simulink model "Simulation_Angle_To_Servo"  (R2020a)
settings: Solver=VariableStepAuto  StartTime=0.0  StopTime=10.0  RelTol=1e-3
values from neighbouring files (symbols this model uses):
  AValues = griddata(data.alpha,data.beta,data.AngleservoA,Alpha,Beta)    [dataToLookupTable.m]
  BValues = griddata(data.alpha,data.beta,data.AngleservoB,Alpha,Beta)    [dataToLookupTable.m]
  CValues = griddata(data.alpha,data.beta,data.AngleservoC,Alpha,Beta)    [dataToLookupTable.m]
settings Model: Creator=vince  LastModifiedBy=vince

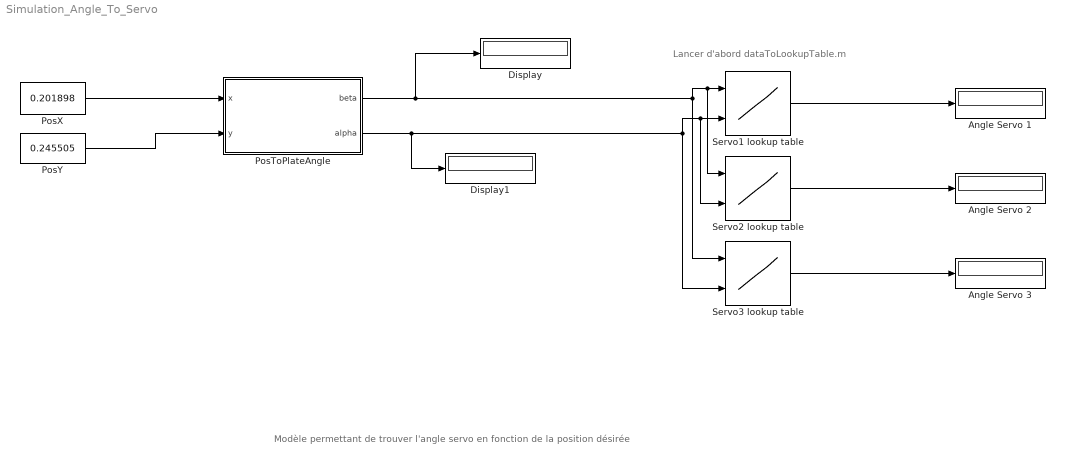
== system Simulation_Angle_To_Servo ==
  note: Modèle permettant de trouver l'angle servo en fonction de la position désirée
  note: Lancer d'abord dataToLookupTable.m
  Angle Servo 1 : Display
  Angle Servo 2 : Display
  Angle Servo 3 : Display
  Display : Display
  Display1 : Display
  PosToPlateAngle : MATLAB Function  TreatAsAtomicUnit=on
  PosX : Constant  Value=0.201898
  PosY : Constant  Value=0.245505
  Servo1 lookup table : Lookup_n-D  BreakpointsSpecification=Even spacing  BreakpointsForDimension1=[1:1801]  BreakpointsForDimension2=[1:176]  BreakpointsForDimension3=[2:316988]  BreakpointsForDimension1FirstPoint=0  BreakpointsForDimension2FirstPoint=0  BreakpointsForDimension1Spacing=0.2  BreakpointsForDimension2Spacing=0.2  IndexSearchMethod=Evenly spaced points  Table=AValues  TableDataTypeStr=Inherit: Inherit from 'Table data'  InterpMethod=Nearest  InternalRulePriority=Speed  OutMin=[3]  OutMax=[3]  OutDataTypeStr=Inherit: Inherit from 'Table data'  RndMeth=Simplest  InputSameDT=on
  Servo2 lookup table : Lookup_n-D  BreakpointsSpecification=Even spacing  BreakpointsForDimension1=[1:1801]  BreakpointsForDimension2=[1:176]  BreakpointsForDimension3=[2:316988]  BreakpointsForDimension1FirstPoint=0  BreakpointsForDimension2FirstPoint=0  BreakpointsForDimension1Spacing=0.2  BreakpointsForDimension2Spacing=0.2  IndexSearchMethod=Evenly spaced points  Table=BValues  TableDataTypeStr=Inherit: Inherit from 'Table data'  InterpMethod=Nearest  InternalRulePriority=Speed  OutMin=[3]  OutMax=[3]  OutDataTypeStr=Inherit: Inherit from 'Table data'  RndMeth=Simplest  InputSameDT=on
  Servo3 lookup table : Lookup_n-D  BreakpointsSpecification=Even spacing  BreakpointsForDimension1=[1:1801]  BreakpointsForDimension2=[1:176]  BreakpointsForDimension3=[2:316988]  BreakpointsForDimension1FirstPoint=0  BreakpointsForDimension2FirstPoint=0  BreakpointsForDimension1Spacing=0.2  BreakpointsForDimension2Spacing=0.2  IndexSearchMethod=Evenly spaced points  Table=CValues  TableDataTypeStr=Inherit: Inherit from 'Table data'  InterpMethod=Nearest  InternalRulePriority=Speed  OutMin=[3]  OutMax=[3]  OutDataTypeStr=Inherit: Inherit from 'Table data'  RndMeth=Simplest  InputSameDT=on
  wires:
  Servo1 lookup table/1 -> Angle Servo 1/1
  PosToPlateAngle/1(beta) -> Display/1, Servo2 lookup table/1, Servo1 lookup table/1, Servo3 lookup table/1
  PosToPlateAngle/2(alpha) -> Display1/1, Servo3 lookup table/2, Servo2 lookup table/2, Servo1 lookup table/2
  Servo2 lookup table/1 -> Angle Servo 2/1
  Servo3 lookup table/1 -> Angle Servo 3/1
  PosX/1 -> PosToPlateAngle/1(x)
  PosY/1 -> PosToPlateAngle/2(y)

== matlab function Simulation_Angle_To_Servo/PosToPlateAngle ==
  data: beta output; x input; alpha output; y input
function [beta,alpha] = PosToPlateAngle(x,y)
toDeg=180/pi;
alpha=asin(sqrt(x^2+y^2))*toDeg;
gamma = atan(y/x)*toDeg;

if (x>0 && y>=0)
    beta=180-abs(gamma);
elseif (x>0 && y<=0)
    beta=180+abs(gamma);
elseif(x<0 && y>=0)
    beta=abs(gamma);
elseif(x<0 && y<=0)
    beta=360-abs(gamma);
elseif(x==0 && y>= 0)
    beta=90;
else
    beta=270;
end
